simulink model "druga_polowa"  (R2018b)
settings: Solver=VariableStepAuto  StartTime=0.0  StopTime=100  RelTol=1e-3
undefined symbols (not defined in the file or in its folder): e0, e1, h, K, N, T
libraries: simulink x1
settings Model: Creator=podstawy  LastModifiedBy=podstawy

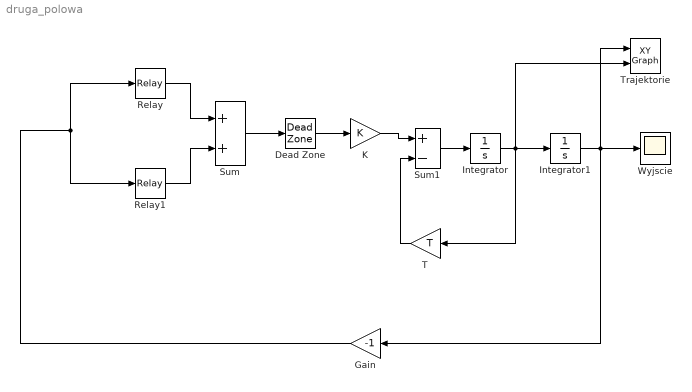
== system druga_polowa ==
  Dead Zone : DeadZone  LowerValue=-N  UpperValue=N  SaturateOnIntegerOverflow=on
  Gain : Gain  Gain=-1
  Integrator : Integrator  InitialCondition=e1
  Integrator1 : Integrator  InitialCondition=e0
  K : Gain  Gain=K
  Relay : Relay  OnSwitchValue=N+h  OffSwitchValue=N
  Relay1 : Relay  OnSwitchValue=-N  OffSwitchValue=-N-h  OnOutputValue=0  OffOutputValue=-1
  Sum : Sum
  Sum1 : Sum  Inputs=+-
  T : Gain  Gain=T
  Trajektorie : simulink/Sinks/XY Graph  xmin=-1  xmax=1  ymin=-1  ymax=1  st=-1
  Wyjscie : Scope
  wires:
  Relay/1 -> Sum/1
  Relay1/1 -> Sum/2
  Sum/1 -> Dead Zone/1
  Dead Zone/1 -> K/1
  K/1 -> Sum1/1
  Sum1/1 -> Integrator/1
  Integrator/1 -> Integrator1/1, T/1, Trajektorie/2
  Integrator1/1 -> Gain/1, Trajektorie/1, Wyjscie/1
  T/1 -> Sum1/2
  Gain/1 -> Relay1/1, Relay/1
